simulink model "ev"  (R2021a)
settings: Solver=ode4  StartTime=0  StopTime=1082  FixedStep=sim_dt  RelTol=1e-3
model workspace (MAT data in the model file):
  T_eff_bp = [-270; -210; -150; -90; -30; 30; 90; 150; 210; 270]
  T_eff_bp_2 = [-270; -210; -150; -90; -30; 30; 90; 150; 210; 270]
  losses_table = [108927.107777 7820.2782368 7820.17609997 7820.2782368 7820.2782368 7820.2782368 7820.2782368 7820.26172359 7820.2782368 9345.38006027 108927.107777 7820.2782368 ... (100 elements, 10x10)]
  losses_table_2 = [108927.107777 7820.2782368 7820.17609997 7820.2782368 7820.2782368 7820.2782368 7820.2782368 7820.26172359 7820.2782368 9345.38006027 108927.107777 7820.2782368 ... (100 elements, 10x10)]
  w_eff_bp = [0; 888.888888889; 1777.77777778; 2666.66666667; 3555.55555556; 4444.44444444; 5333.33333333; 6222.22222222; 7111.11111111; 8000]
  w_eff_bp_2 = [0; 888.888888889; 1777.77777778; 2666.66666667; 3555.55555556; 4444.44444444; 5333.33333333; 6222.22222222; 7111.11111111; 8000]
undefined symbols (not defined in the file): Af, alpha, Bt, C, C_fa, C_free, C_sa_bat, C_sa_uc, Cd, Cmax, Continuous, Crr, DoD, effi, etaFD, etaG, FD, G, gear, Iucmax, m, M1m, M2m, Max, npar, npar_free, npara, nparf, nparfa, nparsa_bat, nparsa_UC, nser, nser_free, nserfa, nsersa_bat, nsersa_UC, Qbat, regenmax, Ri_BP, RL, ro, Rsc, Rsc_A, Rsc_F, Rsc_sa_bat, Rsc_sa_uc, rw, sim_dt, SOC_BP, SoCbatmax, SoCbatmin, SoCucmax, SoCucmin, speed, torque, VinBat, Voc_BP, Vuc, Vuc_fa, Vuc_free ... (+2)
libraries: autolibshared x41, simulink x26, autolibdcdc x13, autolibdatasheetbattery x7, autolibmappedmotor x6, fl_lib x3, nesl_utility x3, spsSupercapacitorLib x3, pid_lib x1
(part 17 of 18)

== system ev/Tesis/HESS/Free/Subsystem/motor speed estimation ==
  vel_m/s : Inport
  Gain : Gain  Gain=1/(rw)
  Scope1 : Scope
  transmission : Product
  motor angular speed : Outport
  wires:
  transmission/1 -> motor angular speed/1, Scope1/1  "motor angular speed"
  [gear_ratio] -> transmission/2
  Gain/1 -> transmission/1  "wheel angular speed"
  vel_m/s/1 -> Gain/1

== system ev/Tesis/HESS/Full_active/Subsystem/motor speed estimation ==
  vel_m/s : Inport
  Gain : Gain  Gain=1/(rw)
  Scope1 : Scope
  transmission : Product
  motor angular speed : Outport
  wires:
  transmission/1 -> motor angular speed/1, Scope1/1  "motor angular speed"
  [gear_ratio] -> transmission/2
  Gain/1 -> transmission/1  "wheel angular speed"
  vel_m/s/1 -> Gain/1

== system ev/Tesis/HESS/semi_active_UC/Subsystem/motor speed estimation ==
  vel_m/s : Inport
  Gain : Gain  Gain=1/(rw)
  Scope1 : Scope
  transmission : Product
  motor angular speed : Outport
  wires:
  transmission/1 -> motor angular speed/1, Scope1/1  "motor angular speed"
  [gear_ratio] -> transmission/2
  Gain/1 -> transmission/1  "wheel angular speed"
  vel_m/s/1 -> Gain/1

== system ev/Tesis/HESS/semi_active_bat/Subsystem/motor speed estimation ==
  vel_m/s : Inport
  Gain : Gain  Gain=1/(rw)
  Scope1 : Scope
  transmission : Product
  motor angular speed : Outport
  wires:
  transmission/1 -> motor angular speed/1, Scope1/1  "motor angular speed"
  [gear_ratio] -> transmission/2
  Gain/1 -> transmission/1  "wheel angular speed"
  vel_m/s/1 -> Gain/1

== matlab function ev/Tesis/HESS/Full active2/MATLAB Function ==
  data: P_batt output; P_req input; P_uc output; V_batt input; V_uc input; SOCb input; SOCuc input; err output
function [P_batt,P_uc,err] = fcn(P_req,V_batt,V_uc,SOCb,SOCuc)


   Vtot=320;
   Ireq=P_req/Vtot;
   Iucmax=300;
   Ibmax=150;
   Iucmin=-300;
   Ibmin=-150;
   Ihessmax=Iucmax+Ibmax;
   Ihessmin=Iucmin+Ibmin;
   SOCbmin=0.2;
   SOCucmin=0.2
   
   if P_req==0 %&& SOCb>SOCbmin && SOCuc>SOCucmin                         %mode 0
       P_batt=0;
       P_uc=0;
       err=0;
   elseif Ireq>Ihessmax
       P_uc=Iucmin*V_uc;
       P_batt=Ibmin*V_batt;
       err=2;
   elseif Ireq<Ihessmin
       P_uc=Iucmax*V_uc;
       P_batt=Ibmax*V_batt;
       err=2;
   elseif P_req>0 && SOCb>=SOCbmin && SOCuc<=SOCucmin                      %mode 1
       P_uc=Iucmin*V_uc;%[A] search the maximum charge current
       P_batt=P_req-P_uc;
       err=1;
   elseif P_req>0 && SOCb>SOCbmin && SOCuc>SOCucmin && Ireq>=Iucmax       %mode 2a
       P_uc=Iucmax*V_uc;
       P_batt=P_req-Iucmax*V_uc;
       err=2;
   elseif P_req>0 && SOCb>SOCbmin && SOCuc>SOCucmin && Ireq<Iucmax       %mode 2b
       P_uc=Ireq*V_uc;
       P_batt=0;
       err=2;
   elseif P_req<0 && SOCb>=SOCbmin && SOCuc<=SOCucmin                      %mode 3
       P_batt=0;
       P_uc=Ireq*V_uc;
       err=3;
   elseif P_req<0 && SOCb<SOCbmin && SOCuc<SOCucmin && Ireq<=Iucmin       %mode 4a
       P_uc=Iucmin*V_uc;
       P_batt=P_req-P_uc;
       err=4;
   elseif P_req<0 && SOCb<SOCbmin && SOCuc<SOCucmin && Ireq>Iucmin       %mode 4b
       P_uc=Ireq*V_uc;
       P_batt=0;
       err=4;
   elseif P_req>0 && SOCb<=SOCbmin && SOCuc<=SOCucmin                      %mode 5
       P_uc=0;
       P_batt=0;
       err=5;
   elseif P_req>0 && SOCb<SOCbmin && SOCuc>SOCucmin                      %mode 6
       P_uc=Ireq*V_uc;
       P_batt=0;
       err=6;
   else
       P_uc=0;
       P_batt=Ireq*V_batt;
       err=-1;
       
       
   end
   


end

== matlab function ev/Tesis/HESS/Full active2/MATLAB Function1 ==
  data: OCV input; I_batt output; Ri input; P input
function I_batt   = fcn(OCV,Ri,P)

%I_batt=(-OCV-sqrt((OCV^2)-(4*(-Ri)*(-P))))/(2*(-Ri));

I_batt=(-(OCV-(OCV^2-4*P*Ri)^(1/2))/(2*Ri));

% I_batt=roots([Ri -OCV P]);
% imIb=imag(I_batt);
% I_batt=min(imIb)
end

== matlab function ev/Tesis/HESS/Full active2/MATLAB Function2 ==
  data: Ri input; Vb output; Ib input; Pmot input
function Vb = fcn(Ri,Ib,Pmot)

Vb=-(((Ri*(Ib^2))+Pmot)/(Ib));


end

== matlab function ev/Tesis/HESS/semi active battery//uc/MATLAB Function ==
  data: Ireq output; Iout output; Preq input; V_bat input; V_uc input; Ibat output; Iuc output; SoCbat input; SoCuc input; err output; stop output; test input; flagpow output; mode output; convDCDC input
function [Ireq,Iout,Ibat,Iuc,err,stop,flagpow,mode] = fcn(Preq,V_bat,V_uc,SoCbat,SoCuc,test,convDCDC)
conDCDC=1;
if V_bat==V_uc
    V_tot=V_bat;
else
    V_tot=V_uc;
end


Ireq=(Preq/V_tot);
Ibatdis=150;
Ibatcha=-150;
Pbatcha=Ibatcha*V_tot*convDCDC;
Pbatdis=Ibatdis*V_tot*convDCDC;
Iucdis=300;
Iuccha=-300;
Puccha=Iuccha*V_tot*conDCDC;
Pucdis=Iucdis*V_tot*conDCDC;


SoCbatmin=0.2;
SoCucmin=0.2;
SoCbatmax=0.85;
SoCucmax=0.95;




   if Preq==0
       mode=0;
   elseif Preq>0
       if Preq<=(Pucdis+Pbatdis)
          if SoCbat<=SoCbatmin
              if SoCuc<=SoCucmin
                  mode=1;
              else
                  if Iucdis>=Ireq
                      mode=2;
                  else
                      mode=3;
                  end
              end
          else
              if SoCuc<=SoCucmin
                  if Ibatdis*convDCDC>=Ireq
                      mode=4;
                  else
                      mode=5;
                  end
              else
                  if test>0
                      if Iucdis*conDCDC>=Ireq
                          mode=6;
                      else
                          mode=7;
                      end
                  elseif test<0
                      if Ibatdis*convDCDC>=Ireq
                          mode=8;
                      else
                          mode=9;
                      end
                  else
                      mode=25;
                  end
              end
          end
       else
           if SoCbat<=SoCbatmin
               if SoCuc<=SoCucmin
                   mode=10;
               else
                   mode=11;
               end
           else
               if SoCuc<=SoCucmin
                   mode=12;
               else
                   mode=13;
               end
           end
       end
   elseif Preq<0
       if Preq>=(Puccha+Pbatcha)
           if SoCuc<=SoCucmax
               if SoCbat<=SoCbatmax
                   if Iuccha*conDCDC>Ireq
                       mode=14;
                   else
                       mode=15;
                   end
               else
                   if Iuccha*conDCDC>Ireq
                       mode=16;
                   else
                       mode=17;
                   end
               end
           else
               if SoCbat<=SoCbatmax
                   if Ibatcha*convDCDC>Ireq
                       mode=18;
                   else
                       mode=19;
                   end
               else
                   mode=20;
               end
           end
       else
           if SoCuc<=SoCucmax
               if SoCbat<=SoCbatmax
                   mode=21;
               else
                   mode=22;
               end
           else
               if SoCbat<=SoCbatmax
                   mode=23;
               else
                   mode=24;
               end
           end
       end
   else
       mode=26;
   end
   
   switch mode
       case 0
           Iuc=0;
           Ibat=0;
           stop=0;
           err=0;
           flagpow=0;           
       case 1
           Iuc=0;
           Ibat=0;
           stop=1;
           err=0;
           flagpow=0;
       case 2
           Iuc=Ireq;
           Ibat=0;
           stop=0;
           err=0;
           flagpow=0;
       case 3
           Iuc=Iucdis*conDCDC;
           Ibat=0;
           stop=0;
           err=0;
           flagpow=1;
       case 4
           Iuc=Ireq-Ibatdis*convDCDC;
           Ibat=Ibatdis*convDCDC;
           stop=0;
           err=0;
           flagpow=0;
       case 5
           Iuc=0;
           Ibat=Ibatdis*convDCDC;
           stop=0;
           err=0;
           flagpow=1;
       case 6
           Iuc=Ireq;
           Ibat=0;
           stop=0;
           err=0;
           flagpow=0;
       case 7
           Iuc=Iucdis*conDCDC;
           Ibat=Ireq-Iucdis*conDCDC;
           stop=0;
           err=0;
           flagpow=0;
       case 8
           Iuc=Ireq-Ibatdis*convDCDC;
           Ibat=Ibatdis*convDCDC;
           stop=0;
           err=0;
           flagpow=0;
       case 9
           Iuc=0;
           Ibat=Ibatdis*convDCDC;
           stop=0;
           err=0;
           flagpow=1;
       case 10
           Iuc=0;
           Ibat=0;
           stop=1;
           err=0;
           flagpow=1;
       case 11
           Iuc=Iucdis*conDCDC;
           Ibat=0;
           stop=0;
           err=0;
           flagpow=1;
       case 12
           Iuc=0;
           Ibat=Ibatdis*convDCDC;
           stop=0;
           err=0;
           flagpow=1;
       case 13
           Iuc=Iucdis*conDCDC;
           Ibat=Ibatdis*convDCDC;
           stop=0;
           err=0;
           flagpow=1;
       case 14
           Iuc=Iuccha*conDCDC;
           Ibat=Ireq-Iuccha*conDCDC;
           stop=0;
           err=0;
           flagpow=0;
       case 15 %mod
           Iuc=0;
           Ibat=Ireq;
           stop=0;
           err=0;
           flagpow=0;
       case 16
           Iuc=Iuccha*conDCDC;
           Ibat=0;
           stop=0;
           err=0;
           flagpow=1;
       case 17
           Iuc=Ireq;
           Ibat=0;
           stop=0;
           err=0;
           flagpow=0;
       case 18
           Iuc=0;
           Ibat=Ibatcha*convDCDC;
           stop=0;
           err=0;
           flagpow=0;
       case 19 %mod
           Iuc=0;
           Ibat=Ireq;
           stop=0;
           err=0;
           flagpow=0;
       case 20
           Iuc=0;
           Ibat=0;
           stop=0;
           err=0;
           flagpow=1;
       case 21
           Iuc=Iuccha*conDCDC;
           Ibat=Ibatcha*convDCDC;
           stop=0;
           err=0;
           flagpow=1;
       case 22
           Iuc=Iuccha*conDCDC;
           Ibat=0;
           stop=0;
           err=0;
           flagpow=1;
       case 23
           Iuc=0;
           Ibat=Ibatcha*convDCDC;
           stop=0;
           err=0;
           flagpow=1;
       case 24
           Iuc=0;
           Ibat=0;
           stop=0;
           err=0;
           flagpow=1;
       case 25 %case when count is 0
           Iuc=0;
           Ibat=0;
           stop=0;
           err=1;
           flagpow=0;
       case 26 %¿? it should not exist
           Iuc=0;
           Ibat=0;
           stop=0;
           err=2;
           flagpow=0;
       otherwise
           Iuc=0;
           Ibat=0;
           stop=0;
           err=3;
           flagpow=0;
           mode=27
   end
   Iuc=Iuc*1;
   Ibat=Ibat*1;
Iout=Iuc+Ibat;

end

== matlab function ev/Tesis/HESS/semi active Bat//Bat/MATLAB Function1 ==
  data: SoCuc input; acurr output; bcurr output; mo1 output; mo2 output; aprev input; bprev input; count output; cprev input; a output; b output; test output
function [acurr,bcurr,mo1,mo2,count,a,b,test] = fcn(SoCuc,aprev,bprev,cprev)

if SoCuc>0.2
    acurr=0;
    mo1=1;
else
    acurr=1;
    mo1=2;
end
if SoCuc>=0.95
    bcurr=1;
    mo2=1;
else
    bcurr=0;
    mo2=2;
end

a=acurr-aprev;
b=bcurr-bprev;


if a==1 || b==1
    count=cprev+a+b;
else
    count=cprev;
end

test=(-1)^(count);

end

== matlab function ev/Tesis/HESS/Full_active/MATLAB Function ==
  data: Ireq output; Iout output; Preq input; V_bat input; V_uc input; Ibat output; Iuc output; SoCbat input; SoCuc input; err output; stop output; test input; flagpow output; mode output; convDCDC input; conDCDC input; Qbat parameter; nparsa_bat parameter; Iucmax parameter; npara parameter; SoCbatmin parameter; SoCucmin parameter; SoCbatmax parameter; SoCucmax parameter; Cmax parameter
function [Ireq,Iout,Ibat,Iuc,err,stop,flagpow,mode] = fcn(Preq,V_bat,V_uc,SoCbat,SoCuc,test,convDCDC,conDCDC,Qbat, nparsa_bat, Iucmax, npara, SoCbatmin, SoCucmin, SoCbatmax, SoCucmax,Cmax)

% if V_bat==V_uc
%     V_tot=V_bat;
% else
%     V_tot=V_uc;
% end

V_tot=320;


Ireq=(Preq/V_tot);

Ibatdis=Qbat*nparsa_bat*Cmax;
Ibatcha=-Qbat*nparsa_bat*Cmax;

Pbatcha=Ibatcha*V_bat;%*convDCDC;
Pbatdis=Ibatdis*V_bat;%*convDCDC;

Iucdis=Iucmax*npara;
Iuccha=-Iucmax*npara;

Puccha=Iuccha*V_uc;%*conDCDC;
Pucdis=Iucdis*V_uc;%*conDCDC;



   if Preq==0
       mode=0;
   elseif Preq>0
       if Preq<=(Pucdis+Pbatdis)
          if SoCbat<=SoCbatmin
              if SoCuc<=SoCucmin
                  mode=1;
              else
                  if Iucdis*convDCDC>=Ireq
                      mode=2;
                  else
                      mode=3;
                  end
              end
          else
              if SoCuc<=SoCucmin
                  if Ibatdis*convDCDC>=Ireq
                      mode=4;
                  else
                      mode=5;
                  end
              elseif SoCuc>0.98
                  if Iucdis*conDCDC>=Ireq
                      mode=27;
                  else
                      mode=28;
                  end
              else
                  if test>0
                      if Ibatdis*convDCDC>=Ireq
                          mode=6;
                      else
                          mode=7;
                      end
                  elseif test<0
                      if Ibatdis*convDCDC>=Ireq
                          mode=8;
                      else
                          mode=9;
                      end
                  else
                      mode=25;
                  end
              end
          end
       else
           if SoCbat<=SoCbatmin
               if SoCuc<=SoCucmin
                   mode=10;
               else
                   mode=11;
               end
           else
               if SoCuc<=SoCucmin
                   mode=12;
               else
                   mode=13;
               end
           end
       end
   elseif Preq<0
       if Preq>=(Puccha+Pbatcha)
           if SoCuc<=SoCucmax
               if SoCbat<=SoCbatmax
                   if Iuccha*conDCDC>Ireq
                       mode=14;
                   else
                       mode=15;
                   end
               else
                   if Iuccha*conDCDC>Ireq
                       mode=16;
                   else
                       mode=17;
                   end
               end
           else
               if SoCbat<=SoCbatmax
                   if Ibatcha*convDCDC>Ireq
                       mode=18;
                   else
                       mode=19;
                   end
               else
                   mode=20;
               end
           end
       else
           if SoCuc<=SoCucmax
               if SoCbat<=SoCbatmax
                   mode=21;
               else
                   mode=22;
               end
           else
               if SoCbat<=SoCbatmax
                   mode=23;
               else
                   mode=24;
               end
           end
       end
   else
       mode=26;
   end
   
   switch mode
       case 0
           Iuc=0;
           Ibat=0;
           stop=0;
           err=0;
           flagpow=0;           
       case 1
           Iuc=0;
           Ibat=0;
           stop=1;
           err=0;
           flagpow=0;
       case 2
           Iuc=Ireq;
           Ibat=0;
           stop=0;
           err=0;
           flagpow=0;
       case 3
           Iuc=Iucdis*conDCDC;
           Ibat=0;
           stop=0;
           err=0;
           flagpow=1;
       case 4
           Iuc=Ireq-Ibatdis*convDCDC;
           Ibat=Ibatdis*convDCDC;
           stop=0;
           err=0;
           flagpow=0;
       case 5
           Iuc=0;
           Ibat=Ibatdis*convDCDC;
           stop=0;
           err=0;
           flagpow=1;
       case 6
           Iuc=0;
           Ibat=Ireq;
           stop=0;
           err=0;
           flagpow=0;
       case 7
           Iuc=Ireq-Ibatdis*convDCDC;
           Ibat=Ibatdis*convDCDC;
           stop=0;
           err=0;
           flagpow=0;
       case 8
           Iuc=-(Ibatdis*convDCDC-Ireq);
           Ibat=Ibatdis*convDCDC;
           stop=0;
           err=0;
           flagpow=0;
       case 9
           Iuc=0;
           Ibat=Ibatdis*convDCDC;
           stop=0;
           err=0;
           flagpow=1;
       case 10
           Iuc=0;
           Ibat=0;
           stop=1;
           err=0;
           flagpow=1;
       case 11
           Iuc=Iucdis*conDCDC;
           Ibat=0;
           stop=0;
           err=0;
           flagpow=1;
       case 12
           Iuc=0;
           Ibat=Ibatdis*convDCDC;
           stop=0;
           err=0;
           flagpow=1;
       case 13
           Iuc=Iucdis*conDCDC;
           Ibat=Ibatdis*convDCDC;
           stop=0;
           err=0;
           flagpow=1;
       case 14
           Iuc=Iuccha*conDCDC;;
           Ibat=Ireq-Iuccha*conDCDC;
           stop=0;
           err=0;
           flagpow=0;
       case 15 %mod
           Iuc=Ireq;
           Ibat=0;
           stop=0;
           err=0;
           flagpow=0;
       case 16
           Iuc=Iuccha*conDCDC;
           Ibat=0;
           stop=0;
           err=0;
           flagpow=1;
       case 17
           Iuc=Ireq;
           Ibat=0;
           stop=0;
           err=0;
           flagpow=0;
       case 18
           Iuc=0;
           Ibat=Ibatcha*convDCDC;
           stop=0;
           err=0;
           flagpow=0;
       case 19 %mod
           Iuc=0;
           Ibat=Ireq;
           stop=0;
           err=0;
           flagpow=0;
       case 20
           Iuc=0;
           Ibat=0;
           stop=0;
           err=0;
           flagpow=1;
       case 21
           Iuc=Iuccha*conDCDC;
           Ibat=Ibatcha*convDCDC;
           stop=0;
           err=0;
           flagpow=1;
       case 22
           Iuc=Iuccha*conDCDC;
           Ibat=0;
           stop=0;
           err=0;
           flagpow=1;
       case 23
           Iuc=0;
           Ibat=Ibatcha*convDCDC;
           stop=0;
           err=0;
           flagpow=1;
       case 24
           Iuc=0;
           Ibat=0;
           stop=0;
           err=0;
           flagpow=1;
       case 25 %case when count is 0
           Iuc=0;
           Ibat=0;
           stop=0;
           err=1;
           flagpow=0;
       case 26 %¿? it should not exist
           Iuc=0;
           Ibat=0;
           stop=0;
           err=2;
           flagpow=0;
       case 27
           Iuc=Ireq;
           Ibat=0;
           stop=0;
           err=2;
           flagpow=0;
       case 28
           Iuc=Iucdis*conDCDC;
           Ibat=Ireq-Iucdis*conDCDC;
           stop=0;
           err=2;
           flagpow=0;
       otherwise
           Iuc=0;
           Ibat=0;
           stop=0;
           err=3;
           flagpow=0;
           mode=29;
   end
   Iuc=Iuc*1;
   Ibat=Ibat*1;
Iout=Iuc+Ibat;

end

== matlab function ev/Tesis/HESS/semi active Bat//Bat/MATLAB Function3 ==
  data: OCV input; I_batt output; Ri input; P input
function I_batt   = fcn(OCV,Ri,P)

%I_batt=(-OCV-sqrt((OCV^2)-(4*(-Ri)*(-P))))/(2*(-Ri));

I_batt=(-(OCV-(OCV^2-4*P*Ri)^(1/2))/(2*Ri));

% I_batt=roots([Ri -OCV P]);
% imIb=imag(I_batt);
% I_batt=min(imIb)
end

== matlab function ev/Tesis/HESS/Full active1/MATLAB Function ==
  data: Ireq output; Iout output; Preq input; V_bat input; V_uc input; Ibat output; Iuc output; SoCbat input; SoCuc input; err output; stop output; test input; flagpow output; mode output; convDCDC input; conDCDC input
function [Ireq,Iout,Ibat,Iuc,err,stop,flagpow,mode] = fcn(Preq,V_bat,V_uc,SoCbat,SoCuc,test,convDCDC,conDCDC)

if V_bat==V_uc
    V_tot=V_bat;
else
    V_tot=V_uc;
end


Ireq=(Preq/V_tot);
Ibatdis=150/1;
Ibatcha=-150/1;
Pbatcha=Ibatcha*V_tot;%*convDCDC;
Pbatdis=Ibatdis*V_tot;%*convDCDC;
Iucdis=300;
Iuccha=-300;
Puccha=Iuccha*V_tot;%*conDCDC;
Pucdis=Iucdis*V_tot;%*conDCDC;


SoCbatmin=0.2;
SoCucmin=0.2;
SoCbatmax=0.85;
SoCucmax=0.95;




   if Preq==0
       mode=0;
   elseif Preq>0
       if Preq<=(Pucdis+Pbatdis)
          if SoCbat<=SoCbatmin
              if SoCuc<=SoCucmin
                  mode=1;
              else
                  if Iucdis*convDCDC>=Ireq
                      mode=2;
                  else
                      mode=3;
                  end
              end
          else
              if SoCuc<=SoCucmin
                  if Ibatdis*convDCDC>=Ireq
                      mode=4;
                  else
                      mode=5;
                  end
              else
                  if test>0
                      if Iucdis*conDCDC>=Ireq
                          mode=6;
                      else
                          mode=7;
                      end
                  elseif test<0
                      if Ibatdis*convDCDC>=Ireq
                          mode=8;
                      else
                          mode=9;
                      end
                  else
                      mode=25;
                  end
              end
          end
       else
           if SoCbat<=SoCbatmin
               if SoCuc<=SoCucmin
                   mode=10;
               else
                   mode=11;
               end
           else
               if SoCuc<=SoCucmin
                   mode=12;
               else
                   mode=13;
               end
           end
       end
   elseif Preq<0
       if Preq>=(Puccha+Pbatcha)
           if SoCuc<=SoCucmax
               if SoCbat<=SoCbatmax
                   if Iuccha*conDCDC>Ireq
                       mode=14;
                   else
                       mode=15;
                   end
               else
                   if Iuccha*conDCDC>Ireq
                       mode=16;
                   else
                       mode=17;
                   end
               end
           else
               if SoCbat<=SoCbatmax
                   if Ibatcha*convDCDC>Ireq
                       mode=18;
                   else
                       mode=19;
                   end
               else
                   mode=20;
               end
           end
       else
           if SoCuc<=SoCucmax
               if SoCbat<=SoCbatmax
                   mode=21;
               else
                   mode=22;
               end
           else
               if SoCbat<=SoCbatmax
                   mode=23;
               else
                   mode=24;
               end
           end
       end
   else
       mode=26;
   end
   
   switch mode
       case 0
           Iuc=0;
           Ibat=0;
           stop=0;
           err=0;
           flagpow=0;           
       case 1
           Iuc=0;
           Ibat=0;
           stop=1;
           err=0;
           flagpow=0;
       case 2
           Iuc=Ireq;
           Ibat=0;
           stop=0;
           err=0;
           flagpow=0;
       case 3
           Iuc=Iucdis*conDCDC;
           Ibat=0;
           stop=0;
           err=0;
           flagpow=1;
       case 4
           Iuc=Ireq-Ibatdis*convDCDC;
           Ibat=Ibatdis*convDCDC;
           stop=0;
           err=0;
           flagpow=0;
       case 5
           Iuc=0;
           Ibat=Ibatdis*convDCDC;
           stop=0;
           err=0;
           flagpow=1;
       case 6
           Iuc=Ireq;
           Ibat=0;
           stop=0;
           err=0;
           flagpow=0;
       case 7
           Iuc=Iucdis*conDCDC;
           Ibat=Ireq-Iucdis*conDCDC;
           stop=0;
           err=0;
           flagpow=0;
       case 8
           Iuc=Ireq-Ibatdis*convDCDC;
           Ibat=Ibatdis*convDCDC;
           stop=0;
           err=0;
           flagpow=0;
       case 9
           Iuc=0;
           Ibat=Ibatdis*convDCDC;
           stop=0;
           err=0;
           flagpow=1;
       case 10
           Iuc=0;
           Ibat=0;
           stop=1;
           err=0;
           flagpow=1;
       case 11
           Iuc=Iucdis*conDCDC;
           Ibat=0;
           stop=0;
           err=0;
           flagpow=1;
       case 12
           Iuc=0;
           Ibat=Ibatdis*convDCDC;
           stop=0;
           err=0;
           flagpow=1;
       case 13
           Iuc=Iucdis*conDCDC;
           Ibat=Ibatdis*convDCDC;
           stop=0;
           err=0;
           flagpow=1;
       case 14
           Iuc=Iuccha*conDCDC;
           Ibat=Ireq-Iuccha*conDCDC;
           stop=0;
           err=0;
           flagpow=0;
       case 15 %mod
           Iuc=0;
           Ibat=Ireq;
           stop=0;
           err=0;
           flagpow=0;
       case 16
           Iuc=Iuccha*conDCDC;
           Ibat=0;
           stop=0;
           err=0;
           flagpow=1;
       case 17
           Iuc=Ireq;
           Ibat=0;
           stop=0;
           err=0;
           flagpow=0;
       case 18
           Iuc=0;
           Ibat=Ibatcha*convDCDC;
           stop=0;
           err=0;
           flagpow=0;
       case 19 %mod
           Iuc=0;
           Ibat=Ireq;
           stop=0;
           err=0;
           flagpow=0;
       case 20
           Iuc=0;
           Ibat=0;
           stop=0;
           err=0;
           flagpow=1;
       case 21
           Iuc=Iuccha*conDCDC;
           Ibat=Ibatcha*convDCDC;
           stop=0;
           err=0;
           flagpow=1;
       case 22
           Iuc=Iuccha*conDCDC;
           Ibat=0;
           stop=0;
           err=0;
           flagpow=1;
       case 23
           Iuc=0;
           Ibat=Ibatcha*convDCDC;
           stop=0;
           err=0;
           flagpow=1;
       case 24
           Iuc=0;
           Ibat=0;
           stop=0;
           err=0;
           flagpow=1;
       case 25 %case when count is 0
           Iuc=0;
           Ibat=0;
           stop=0;
           err=1;
           flagpow=0;
       case 26 %¿? it should not exist
           Iuc=0;
           Ibat=0;
           stop=0;
           err=2;
           flagpow=0;
       otherwise
           Iuc=0;
           Ibat=0;
           stop=0;
           err=3;
           flagpow=0;
           mode=27;
   end
   Iuc=Iuc*1;
   Ibat=Ibat*1;
Iout=Iuc+Ibat;

end

== matlab function ev/Tesis/HESS/Full active1/MATLAB Function1 ==
  data: SoCuc input; acurr output; bcurr output; mo1 output; mo2 output; aprev input; bprev input; count output; cprev input; a output; b output; test output
function [acurr,bcurr,mo1,mo2,count,a,b,test] = fcn(SoCuc,aprev,bprev,cprev)

if SoCuc>0.4
    acurr=0;
    mo1=1;
else
    acurr=1;
    mo1=2;
end
if SoCuc>=1
    bcurr=1;
    mo2=1;
else
    bcurr=0;
    mo2=2;
end

a=acurr-aprev;
b=bcurr-bprev;


if a==1 || b==1
    count=cprev+a+b;
else
    count=cprev;
end

test=(-1)^(count);

end

== matlab function ev/Tesis/HESS/Full active1/MATLAB Function2 ==
  data: Ireq input; Vcons output; Inew output; const output; Vuc input; Vconst input
function [Vcons,Inew,const] = fcn(Ireq,Vuc,Vconst)

Inew=Ireq*Vuc/Vconst;
Vcons=Vconst;
const=Vuc/Vconst;

end

== matlab function ev/Tesis/HESS/Full active3/MATLAB Function ==
  data: Ireq output; Iout output; Preq input; V_bat input; V_uc input; Ibat output; Iuc output; SoCbat input; SoCuc input; err output; stop output; test input; flagpow output; mode output; convDCDC input; conDCDC input
function [Ireq,Iout,Ibat,Iuc,err,stop,flagpow,mode] = fcn(Preq,V_bat,V_uc,SoCbat,SoCuc,test,convDCDC,conDCDC)

if V_bat==V_uc
    V_tot=V_bat;
else
    V_tot=V_uc;
end


Ireq=(Preq/V_tot);
Ibatdis=150/3;
Ibatcha=-150/3;
Pbatcha=Ibatcha*V_tot;%*convDCDC;
Pbatdis=Ibatdis*V_tot;%*convDCDC;
Iucdis=300;
Iuccha=-300;
Puccha=Iuccha*V_tot;%*conDCDC;
Pucdis=Iucdis*V_tot;%*conDCDC;


SoCbatmin=0.2;
SoCucmin=0.2;
SoCbatmax=0.85;
SoCucmax=0.95;




   if Preq==0
       mode=0;
   elseif Preq>0
       if Preq<=(Pucdis+Pbatdis)
          if SoCbat<=SoCbatmin
              if SoCuc<=SoCucmin
                  mode=1;
              else
                  if Iucdis*conDCDC>=Ireq
                      mode=2;
                  else
                      mode=3;
                  end
              end
          else
              if SoCuc<=SoCucmin
                  if Ibatdis*convDCDC>=Ireq
                      mode=4;
                  else
                      mode=5;
                  end
              else
                  if test>0
                      if Iucdis*conDCDC>=Ireq
                          mode=6;
                      else
                          mode=7;
                      end
                  elseif test<0
                      if Ibatdis*convDCDC>=Ireq
                          mode=8;
                      else
                          mode=9;
                      end
                  else
                      mode=25;
                  end
              end
          end
       else
           if SoCbat<=SoCbatmin
               if SoCuc<=SoCucmin
                   mode=10;
               else
                   mode=11;
               end
           else
               if SoCuc<=SoCucmin
                   mode=12;
               else
                   mode=13;
               end
           end
       end
   elseif Preq<0
       if Preq>=(Puccha+Pbatcha)
           if SoCuc<=SoCucmax
               if SoCbat<=SoCbatmax
                   if Iuccha*conDCDC>Ireq
                       mode=14;
                   else
                       mode=15;
                   end
               else
                   if Iuccha*conDCDC>Ireq
                       mode=16;
                   else
                       mode=17;
                   end
               end
           else
               if SoCbat<=SoCbatmax
                   if Ibatcha*convDCDC>Ireq
                       mode=18;
                   else
                       mode=19;
                   end
               else
                   mode=20;
               end
           end
       else
           if SoCuc<=SoCucmax
               if SoCbat<=SoCbatmax
                   mode=21;
               else
                   mode=22;
               end
           else
               if SoCbat<=SoCbatmax
                   mode=23;
               else
                   mode=24;
               end
           end
       end
   else
       mode=26;
   end
   
   switch mode
       case 0
           Iuc=0;
           Ibat=0;
           stop=0;
           err=0;
           flagpow=0;           
       case 1
           Iuc=0;
           Ibat=0;
           stop=1;
           err=0;
           flagpow=0;
       case 2
           Iuc=Ireq;
           Ibat=0;
           stop=0;
           err=0;
           flagpow=0;
       case 3
           Iuc=Iucdis*conDCDC;
           Ibat=0;
           stop=0;
           err=0;
           flagpow=1;
       case 4
           Iuc=Ireq-Ibatdis*convDCDC;
           Ibat=Ibatdis*convDCDC;
           stop=0;
           err=0;
           flagpow=0;
       case 5
           Iuc=0;
           Ibat=Ibatdis*convDCDC;
           stop=0;
           err=0;
           flagpow=1;
       case 6
           Iuc=Ireq;
           Ibat=0;
           stop=0;
           err=0;
           flagpow=0;
       case 7
           Iuc=Iucdis*conDCDC;
           Ibat=Ireq-Iucdis*conDCDC;
           stop=0;
           err=0;
           flagpow=0;
       case 8
           Iuc=Ireq-Ibatdis*convDCDC;
           Ibat=Ibatdis*convDCDC;
           stop=0;
           err=0;
           flagpow=0;
       case 9
           Iuc=0;
           Ibat=Ibatdis*convDCDC;
           stop=0;
           err=0;
           flagpow=1;
       case 10
           Iuc=0;
           Ibat=0;
           stop=1;
           err=0;
           flagpow=1;
       case 11
           Iuc=Iucdis*conDCDC;
           Ibat=0;
           stop=0;
           err=0;
           flagpow=1;
       case 12
           Iuc=0;
           Ibat=Ibatdis*convDCDC;
           stop=0;
           err=0;
           flagpow=1;
       case 13
           Iuc=Iucdis*conDCDC;
           Ibat=Ibatdis*convDCDC;
           stop=0;
           err=0;
           flagpow=1;
       case 14
           Iuc=Iuccha*conDCDC;
           Ibat=Ireq-Iuccha*conDCDC;
           stop=0;
           err=0;
           flagpow=0;
       case 15 %mod
           Iuc=0;
           Ibat=Ireq;
           stop=0;
           err=0;
           flagpow=0;
       case 16
           Iuc=Iuccha*conDCDC;
           Ibat=0;
           stop=0;
           err=0;
           flagpow=1;
       case 17
           Iuc=Ireq;
           Ibat=0;
           stop=0;
           err=0;
           flagpow=0;
       case 18
           Iuc=0;
           Ibat=Ibatcha*convDCDC;
           stop=0;
           err=0;
           flagpow=0;
       case 19 %mod
           Iuc=0;
           Ibat=Ireq;
           stop=0;
           err=0;
           flagpow=0;
       case 20
           Iuc=0;
           Ibat=0;
           stop=0;
           err=0;
           flagpow=1;
       case 21
           Iuc=Iuccha*conDCDC;
           Ibat=Ibatcha*convDCDC;
           stop=0;
           err=0;
           flagpow=1;
       case 22
           Iuc=Iuccha*conDCDC;
           Ibat=0;
           stop=0;
           err=0;
           flagpow=1;
       case 23
           Iuc=0;
           Ibat=Ibatcha*convDCDC;
           stop=0;
           err=0;
           flagpow=1;
       case 24
           Iuc=0;
           Ibat=0;
           stop=0;
           err=0;
           flagpow=1;
       case 25 %case when count is 0
           Iuc=0;
           Ibat=0;
           stop=0;
           err=1;
           flagpow=0;
       case 26 %¿? it should not exist
           Iuc=0;
           Ibat=0;
           stop=0;
           err=2;
           flagpow=0;
       otherwise
           Iuc=0;
           Ibat=0;
           stop=0;
           err=3;
           flagpow=0;
           mode=27
   end
   Iuc=Iuc*1;
   Ibat=Ibat*1;
Iout=Iuc+Ibat;

end

== matlab function ev/Tesis/HESS/Full active3/MATLAB Function1 ==
  data: SoCuc input; acurr output; bcurr output; mo1 output; mo2 output; aprev input; bprev input; count output; cprev input; a output; b output; test output
function [acurr,bcurr,mo1,mo2,count,a,b,test] = fcn(SoCuc,aprev,bprev,cprev)

if SoCuc>0.2
    acurr=0;
    mo1=1;
else
    acurr=1;
    mo1=2;
end
if SoCuc>=0.95
    bcurr=1;
    mo2=1;
else
    bcurr=0;
    mo2=2;
end

a=acurr-aprev;
b=bcurr-bprev;


if a==1 || b==1
    count=cprev+a+b;
else
    count=cprev;
end

test=(-1)^(count);

end

== matlab function ev/Tesis/HESS/Full active3/MATLAB Function2 ==
  data: Ireq input; Vcons output; Inew output; const output; Vuc input; Vconst input
function [Vcons,Inew,const] = fcn(Ireq,Vuc,Vconst)

Inew=Ireq*Vuc/Vconst;
Vcons=Vconst;
const=Vuc/Vconst;

end

== matlab function ev/Tesis/HESS/Full active3/MATLAB Function3 ==
  data: OCV input; I_batt output; Ri input; P input
function I_batt   = fcn(OCV,Ri,P)

%I_batt=(-OCV-sqrt((OCV^2)-(4*(-Ri)*(-P))))/(2*(-Ri));

I_batt=(-(OCV-(OCV^2-4*P*Ri)^(1/2))/(2*Ri));

% I_batt=roots([Ri -OCV P]);
% imIb=imag(I_batt);
% I_batt=min(imIb)
end

== matlab function ev/Tesis/HESS/Full active3/MATLAB Function4 ==
  data: Ri input; Vb output; Ib input; Pmot input
function Vb = fcn(Ri,Ib,Pmot)

Vb=-(((Ri*(Ib^2))+Pmot)/(Ib));


end

== matlab function ev/Tesis/HESS/semi active battery//uc/MATLAB Function1 ==
  data: SoCuc input; acurr output; bcurr output; mo1 output; mo2 output; aprev input; bprev input; count output; cprev input; a output; b output; test output
function [acurr,bcurr,mo1,mo2,count,a,b,test] = fcn(SoCuc,aprev,bprev,cprev)

if SoCuc>0.2
    acurr=0;
    mo1=1;
else
    acurr=1;
    mo1=2;
end
if SoCuc>=0.95
    bcurr=1;
    mo2=1;
else
    bcurr=0;
    mo2=2;
end

a=acurr-aprev;
b=bcurr-bprev;


if a==1 || b==1
    count=cprev+a+b;
else
    count=cprev;
end

test=(-1)^(count);

end

== matlab function ev/Tesis/HESS/semi active battery//uc/MATLAB Function2 ==
  data: Ireq input; Vcons output; Inew output; const output; Vuc input; Vconst input
function [Vcons,Inew,const] = fcn(Ireq,Vuc,Vconst)

Inew=Ireq*Vuc/Vconst;
Vcons=Vconst;
const=Vuc/Vconst;

end

== matlab function ev/Tesis/HESS/semi active battery//uc/MATLAB Function3 ==
  data: OCV input; I_batt output; Ri input; P input
function I_batt   = fcn(OCV,Ri,P)

%I_batt=(-OCV-sqrt((OCV^2)-(4*(-Ri)*(-P))))/(2*(-Ri));

I_batt=(-(OCV-(OCV^2-4*P*Ri)^(1/2))/(2*Ri));

% I_batt=roots([Ri -OCV P]);
% imIb=imag(I_batt);
% I_batt=min(imIb)
end

== matlab function ev/Tesis/HESS/semi active battery//uc/MATLAB Function4 ==
  data: Ri input; Vb output; Ib input; Pmot input
function Vb = fcn(Ri,Ib,Pmot)

Vb=-(((Ri*(Ib^2))+Pmot)/(Ib));


end

== matlab function ev/Tesis/HESS/semi active Bat//Bat/MATLAB Function4 ==
  data: Ri input; Vb output; Ib input; Pmot input
function Vb = fcn(Ri,Ib,Pmot)

Vb=-(((Ri*(Ib^2))+Pmot)/(Ib));


end

== matlab function ev/Tesis/HESS/semi active Bat//Bat/MATLAB Function5 ==
  data: OCV input; I_batt output; Ri input; data input; P input
function I_batt   = fcn(OCV,Ri,data, P)

%I_batt=(-OCV-sqrt((OCV^2)-(4*(-Ri)*(-P))))/(2*(-Ri));

I_batt=(-(OCV-(OCV^2-4*P*Ri)^(1/2))/(2*Ri));

% I_batt=roots([Ri -OCV P]);
% imIb=imag(I_batt);
% I_batt=min(imIb)
end

== matlab function ev/Tesis/HESS/battery model limited/MATLAB Function ==
  data: OCV input; I_batt output; Ri input; P input
function I_batt   = fcn(OCV,Ri,P)

%I_batt=(-OCV-sqrt((OCV^2)-(4*(-Ri)*(-P))))/(2*(-Ri));

I_batt=(-(OCV-(OCV^2-4*P*Ri)^(1/2))/(2*Ri));

% I_batt=roots([Ri -OCV P]);
% imIb=imag(I_batt);
% I_batt=min(imIb)
end

== matlab function ev/Tesis/HESS/semi active Bat//Bat/MATLAB Function6 ==
  data: Ri input; Vb output; Ib input; Pmot input
function Vb = fcn(Ri,Ib,Pmot)

Vb=-(((Ri*(Ib^2))+Pmot)/(Ib));


end

== matlab function ev/Tesis/HESS/Full_active/MATLAB Function1 ==
  data: SoCuc input; acurr output; bcurr output; mo1 output; mo2 output; aprev input; bprev input; count output; cprev input; a output; b output; test output; counta output; countb output; cpreva input; cprevb input; countc output
function [acurr,bcurr,mo1,mo2,count,a,b,test,counta,countb,countc] = fcn(SoCuc,aprev,bprev,cprev,cpreva,cprevb)

if SoCuc>=0.2
    acurr=0;
    mo1=1;
else
    acurr=1;
    mo1=2;
end
if SoCuc>=0.9
    bcurr=1;
    mo2=1;
else
    bcurr=0;
    mo2=2;
end

a=acurr-aprev;
b=bcurr-bprev;




if a==1 || b==1
%     count=cprev+a+b;
    counta=cpreva+a;
    countb=cprevb+b;
else
%     count=cprev;
    counta=cpreva;
    countb=cprevb;
end
countc=countb-counta;

if countc>0
    count=2;
else 
    count=1;
end

test=(-1)^(count);

end

== matlab function ev/Tesis/HESS/Full_active/MATLAB Function3 ==
  data: Id output; Vo input; Vd input; eff input; Po input; Pd output; Io output
function [Id,Pd,Io]  = fcn(Vo,Vd,eff, Po)

if Po>0
    Pd=Po;
    Id=Pd/Vd;
    Io=Po/Vo;
elseif Po<0
    Pd=Po;
    Id=Pd/Vd;
    Io=Po/Vo;
else
    Pd=Po;
    Id=Pd/Vd;
    Io=Po/Vo;
end
   

end

== matlab function ev/Tesis/HESS/Full active4/MATLAB Function ==
  data: Ireq output; Pout output; Preq input; V_bat input; V_uc input; Pbat output; Puc output; SoCbat input; SoCuc input; err output; stop output; test input; flagpow output; mode output
function [Ireq,Pout,Pbat,Puc,err,stop,flagpow,mode] = fcn(Preq,V_bat,V_uc,SoCbat,SoCuc,test)

if V_bat==V_uc
    V_tot=V_bat;
else
    V_tot=V_uc;
end


Ireq=(Preq/V_tot);
Ibatdis=208;
Ibatcha=-208;
Pbatcha=Ibatcha*V_bat;%*convDCDC;
Pbatdis=Ibatdis*V_bat;%*convDCDC;
Iucdis=140*4;
Iuccha=-140*4;
Puccha=Iuccha*V_uc;%*conDCDC;
Pucdis=Iucdis*V_uc;%*conDCDC;


SoCbatmin=0.2;
SoCucmin=0.2;
SoCbatmax=0.85;
SoCucmax=0.95;




   if Preq==0
       mode=0;
   elseif Preq>0
       if Preq<=(Pucdis+Pbatdis)
          if SoCbat<=SoCbatmin
              if SoCuc<=SoCucmin
                  mode=1;
              else
                  if Pucdis>=Preq
                      mode=2;
                  else
                      mode=3;
                  end
              end
          else
              if SoCuc<=SoCucmin
                  if Pbatdis>=Preq
                      mode=4;
                  else
                      mode=5;
                  end
              else
                  if test>0
                      if Pucdis>=Preq
                          mode=6;
                      else
                          mode=7;
                      end
                  elseif test<0
                      if Pbatdis>=Preq
                          mode=8;
                      else
                          mode=9;
                      end
                  else
                      mode=25;
                  end
              end
          end
       else
           if SoCbat<=SoCbatmin
               if SoCuc<=SoCucmin
                   mode=10;
               else
                   mode=11;
               end
           else
               if SoCuc<=SoCucmin
                   mode=12;
               else
                   mode=13;
               end
           end
       end
   elseif Preq<0
       if Preq>=(Puccha+Pbatcha)
           if SoCuc<=SoCucmax
               if SoCbat<=SoCbatmax
                   if Puccha>Preq
                       mode=14;
                   else
                       mode=15;
                   end
               else
                   if Puccha>Preq
                       mode=16;
                   else
                       mode=17;
                   end
               end
           else
               if SoCbat<=SoCbatmax
                   if Pbatcha>Preq
                       mode=18;
                   else
                       mode=19;
                   end
               else
                   mode=20;
               end
           end
       else
           if SoCuc<=SoCucmax
               if SoCbat<=SoCbatmax
                   mode=21;
               else
                   mode=22;
               end
           else
               if SoCbat<=SoCbatmax
                   mode=23;
               else
                   mode=24;
               end
           end
       end
   else
       mode=26;
   end
   
   switch mode
       case 0
           Puc=0;
           Pbat=0;
           stop=0;
           err=0;
           flagpow=0;           
       case 1
           Puc=0;
           Pbat=0;
           stop=1;
           err=0;
           flagpow=0;
       case 2
           Puc=Preq;
           Pbat=0;
           stop=0;
           err=0;
           flagpow=0;
       case 3
           Puc=Pucdis;
           Pbat=0;
           stop=0;
           err=0;
           flagpow=1;
       case 4
           Puc=Preq-Pbatdis;
           Pbat=Pbatdis;
           stop=0;
           err=0;
           flagpow=0;
       case 5
           Puc=0;
           Pbat=Pbatdis;
           stop=0;
           err=0;
           flagpow=1;
       case 6
           Puc=Preq;
           Pbat=0;
           stop=0;
           err=0;
           flagpow=0;
       case 7
           Puc=Pucdis;
           Pbat=Preq-Pucdis;
           stop=0;
           err=0;
           flagpow=0;
       case 8
           Puc=Preq-Pbatdis;
           Pbat=Pbatdis;
           stop=0;
           err=0;
           flagpow=0;
       case 9
           Puc=0;
           Pbat=Pbatdis;
           stop=0;
           err=0;
           flagpow=1;
       case 10
           Puc=0;
           Pbat=0;
           stop=1;
           err=0;
           flagpow=1;
       case 11
           Puc=Pucdis;
           Pbat=0;
           stop=0;
           err=0;
           flagpow=1;
       case 12
           Puc=0;
           Pbat=Pbatdis;
           stop=0;
           err=0;
           flagpow=1;
       case 13
           Puc=Pucdis;
           Pbat=Pbatdis;
           stop=0;
           err=0;
           flagpow=1;
       case 14
           Puc=Puccha;
           Pbat=Preq-Puccha;
           stop=0;
           err=0;
           flagpow=0;
       case 15 %mod
           Puc=0;
           Pbat=Preq;
           stop=0;
           err=0;
           flagpow=0;
       case 16
           Puc=Puccha;
           Pbat=0;
           stop=0;
           err=0;
           flagpow=1;
       case 17
           Puc=Preq;
           Pbat=0;
           stop=0;
           err=0;
           flagpow=0;
       case 18
           Puc=0;
           Pbat=Pbatcha;
           stop=0;
           err=0;
           flagpow=0;
       case 19 %mod
           Puc=0;
           Pbat=Preq;
           stop=0;
           err=0;
           flagpow=0;
       case 20
           Puc=0;
           Pbat=0;
           stop=0;
           err=0;
           flagpow=1;
       case 21
           Puc=Puccha;
           Pbat=Pbatcha;
           stop=0;
           err=0;
           flagpow=1;
       case 22
           Puc=Puccha;
           Pbat=0;
           stop=0;
           err=0;
           flagpow=1;
       case 23
           Puc=0;
           Pbat=Pbatcha;
           stop=0;
           err=0;
           flagpow=1;
       case 24
           Puc=0;
           Pbat=0;
           stop=0;
           err=0;
           flagpow=1;
       case 25 %case when count is 0
           Puc=0;
           Pbat=0;
           stop=0;
           err=1;
           flagpow=0;
       case 26 %¿? it should not exist
           Puc=0;
           Pbat=0;
           stop=0;
           err=2;
           flagpow=0;
       otherwise
           Puc=0;
           Pbat=0;
           stop=0;
           err=3;
           flagpow=0;
           mode=27;
   end
   Puc=Puc*1;
   Pbat=Pbat*1;
Pout=Puc+Pbat;

end

== matlab function ev/Tesis/HESS/Full active4/MATLAB Function1 ==
  data: SoCuc input; acurr output; bcurr output; mo1 output; mo2 output; aprev input; bprev input; count output; cprev input; a output; b output; test output
function [acurr,bcurr,mo1,mo2,count,a,b,test] = fcn(SoCuc,aprev,bprev,cprev)

if SoCuc>0.4
    acurr=0;
    mo1=1;
else
    acurr=1;
    mo1=2;
end
if SoCuc>=1
    bcurr=1;
    mo2=1;
else
    bcurr=0;
    mo2=2;
end

a=acurr-aprev;
b=bcurr-bprev;


if a==1 || b==1
    count=cprev+a+b;
else
    count=cprev;
end

test=(-1)^(count);

end

== matlab function ev/Tesis/HESS/Full_active/MATLAB Function5 ==
  data: Id output; Vo input; Vd input; eff input; Po input; Pd output; Io output
function [Id,Pd,Io]  = fcn(Vo,Vd,eff, Po)

if Po>0
    Pd=Po;
    Id=Pd/Vd;
    Io=Po/Vo;
elseif Po<0
    Pd=Po;
    Id=Pd/Vd;
    Io=Po/Vo;
else
    Pd=Po;
    Id=Pd/Vd;
    Io=Po/Vo;
end
   

end
